simulink model "MotorX_PlantX"  (R2016b)
settings: Solver=VariableStepAuto  StartTime=0.0  StopTime=10.0  RelTol=1e-3
settings Model: Creator=ProBook  LastModifiedBy=ProBook
settings OptimizationCC: DefaultParameterBehavior=Inlined
settings DebuggingCC: InitInArrayFormatMsg=none
settings SFSimCC: SimUseLocalCustomCode=on
settings RTWCC: RTWUseLocalCustomCode=on

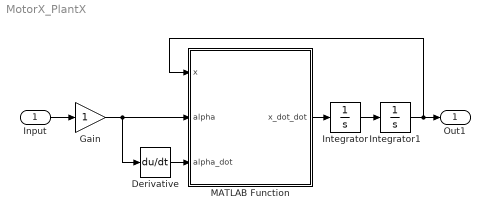
== system MotorX_PlantX ==
  Input : Inport
  Derivative : Derivative
  Gain : Gain
  Integrator : Integrator
  Integrator1 : Integrator
  MATLAB Function : MATLAB Function  TreatAsAtomicUnit=on
  Out1 : Outport
  wires:
  Integrator1/1 -> MATLAB Function/1(x), Out1/1
  MATLAB Function/1(x_dot_dot) -> Integrator/1
  Integrator/1 -> Integrator1/1
  Gain/1 -> Derivative/1, MATLAB Function/2(alpha)
  Derivative/1 -> MATLAB Function/3(alpha_dot)
  Input/1 -> Gain/1

== matlab function MotorX_PlantX/MATLAB Function ==
  data: x input; alpha input; x_dot_dot output; alpha_dot input
function x_dot_dot  = fcn(x,alpha,alpha_dot)
g = 9.81;
B = 5/7;
x_dot_dot = (B)*(x*(alpha_dot^2)) - (B)*g*sin(alpha);
